simulink model "Linear_Controller_Trajectory_Tracking"  (R2020b)
settings: Solver=VariableStepAuto  StartTime=0.0  StopTime=10.0  RelTol=1e-3
settings Model: Creator=24365  LastModifiedBy=24365

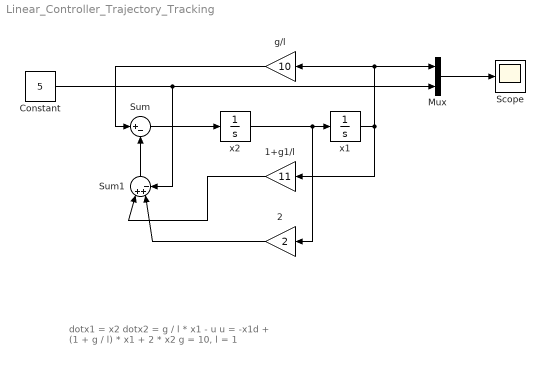
== system Linear_Controller_Trajectory_Tracking ==
  note: dotx1 = x2
      | dotx2 = g / l * x1 - u
      | u = -x1d + (1 + g / l) * x1 + 2 * x2
      | g = 10, l = 1
  1+g1/l : Gain  Gain=11
  2 : Gain  Gain=2
  Constant : Constant  Value=5
  Mux : Mux  Inputs=2
  Scope : Scope
  Sum : Sum  Inputs=|+-
  Sum1 : Sum  Inputs=|++-
  g/l : Gain  Gain=10
  x1 : Integrator
  x2 : Integrator
  wires:
  x2/1 -> 2/1, x1/1
  x1/1 -> Mux/1, g/l/1, 1+g1/l/1
  Sum/1 -> x2/1
  g/l/1 -> Sum/1
  Constant/1 -> Mux/2, Sum1/3
  1+g1/l/1 -> Sum1/1
  2/1 -> Sum1/2
  Mux/1 -> Scope/1
  Sum1/1 -> Sum/2
